simulink model "project_simulink"  (R2024b)
settings: Solver=VariableStepAuto  StartTime=0.0  StopTime=50  RelTol=1e-3
values from neighbouring files (symbols this model uses):
  K2 = -rho_air*Cx*A_front*(v0+v_w0)    (= -14.95725)    [project.m]
  m_star = J_M*(tau_1*tau_2/Rw)^2+4*J_wheel/(Rw^2)+M    (= 1536.32653061)    [project.m]    (also in project_section_1.m)
  r_gen = r_star + C_RR*k_RR*M*g + rho_air*Cx*A_front*(v0 + v_w0)    (= 15.0683126531)    [project.m]    (also in project_section_1.m)
  ratio = Rw/(tau_2*tau_1)    (= 0.116666666667)    [project.m]    (also in project_section_1.m)
settings Model: Creator=Virgile  LastModifiedBy=Virgile

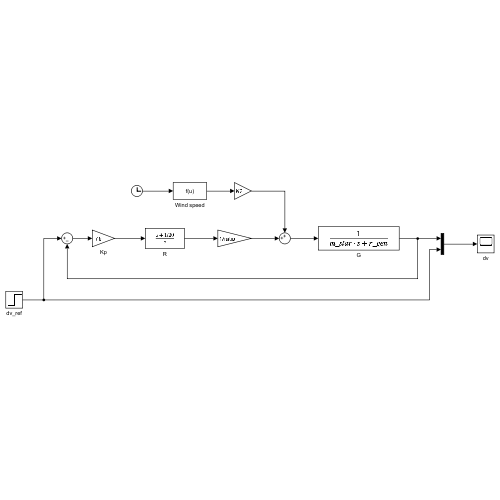
[thumbnail: Simulink's stored preview of the top-level diagram]
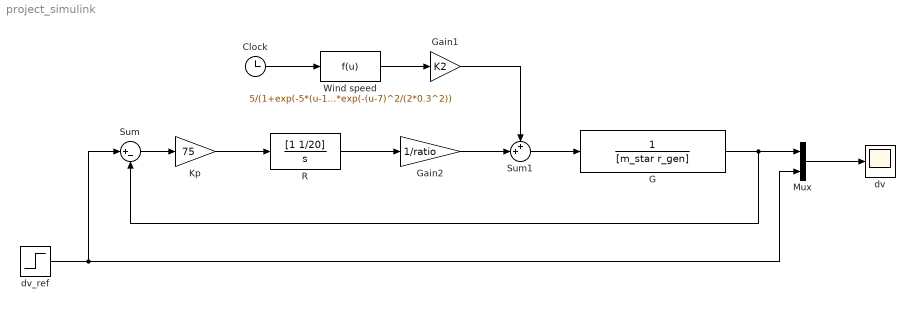
== system project_simulink ==
  Clock : Clock
  G : TransferFcn  Denominator=[m_star r_gen]
  Gain1 : Gain  Gain=K2
  Gain2 : Gain  Gain=1/ratio
  Kp : Gain  Gain=75
  Mux : Mux  Inputs=2
  R : TransferFcn  Numerator=[1 1/20]  Denominator=[1 0]
  Sum : Sum  Inputs=|+-
  Sum1 : Sum  Inputs=++|
  Wind speed : Fcn  Expr=5/(1+exp(-5*(u-1.5)))+4*exp(-(u-7)^2/(2*0.3^2))
  dv : Scope
  dv_ref : Step  SampleTime=0.1
  wires:
  G/1 -> Sum/2, Mux/1
  Sum/1 -> Kp/1
  Kp/1 -> R/1
  R/1 -> Gain2/1
  Sum1/1 -> G/1
  Gain2/1 -> Sum1/2
  Gain1/1 -> Sum1/1
  Clock/1 -> Wind speed/1
  Wind speed/1 -> Gain1/1
  Mux/1 -> dv/1
  dv_ref/1 -> Sum/1, Mux/2
